simulink model "Control_test"  (R2014b)
settings: Solver=FixedStepDiscrete  StartTime=0.0  StopTime=Inf  FixedStep=0.001  RelTol=1e-3
PostLoadFcn:
  | , if any(exist('dsrtsu_mdlpostloadfcn', 'file') == [2, 3, 6]), try dsrtsu_mdlpostloadfcn('Execute', bdroot); catch fprintf('Error in PostLoadFcn (dsrtsu_mdlpostloadfcn) for model "%s":\n %s\n', bdroot, lasterr); end, end,
undefined symbols (not defined in the file or in its folder): dtLocal, slcm
libraries: rtican x163, simulink x14
(part 32 of 34)

== system Control_test/InputProcessing/VehicleCanProcessing/TCS3 ==
  Bus Creator : BusCreator  Inputs=17
  L_TCS3 : rtican/RTICAN Receive (RX)   Reserved1=[]  Reserved2=[]  Reserved3=[]  Reserved4=[]  SfcnMessage=[]  Msg_Struct=[]  BoardTypeNo=[]  BoardNo=[]  ChannelNo=[]  Parameters=[]  DialogFcn=[]  UnitName=[]  Revision=[]  UnitValues=[]  DSProperties=struct('RTI',struct('Version',uint32(5),'BlockType',struct('isSLSource',uint8(1),'isSLSink',uint8(1),'isHWSource',uint8(0),'isHWSink',uint8(0),'isSetup',uint8(0),'isInline',uint8(1),'isNonInline',uint8(0),'isInterrupt',uint8(0),'isChannelwise',uint8(0)),'IOBoardType','RTICAN','UnitType','MESSAGE','Identifier','RX','DialogType','MSVC','BlockSet','RTICAN','SlaveProcessor','CAN'))  RTIBlockInterface=struct('OutputPortsWidth',int32([1 1 1 1 1 1 1 1 1 1 1 1 1 1 1 1 1]),'OutputPortsActive',[1 1 1 1 1 1 1 1 1 1 1 1 1 1 1 1 1],'OutputPortsName',{{'aBasis','BrakeLight','DCEnable','AliveCounterTCS','MinGear','MaxGear','ACCReqLim','TQI_ACC','ACCEL_REF_ACC','ACCEnable','DriverOverride','StandStill','CheckSum_TCS3','ACC_EQUIP','PBRAKE_ACT','ACC_REQ','DriverBraking'}},'OutputPortsDataType',{{'SS_DOUBLE','SS_DOUBLE','SS_DOUBLE','SS_DOUBLE','SS_DOUBLE','SS_DOUBLE','SS_DOUBLE','SS_DOUBLE','SS_DOUBLE','SS_DOUBLE','SS_DOUBLE','SS_DOUBLE','SS_DOUBLE','SS_DOUBLE','SS_DOUBLE','SS_DOUBLE','SS_DOUBLE'}},'OutputPortsLabel',{{'aBasis','BrakeLight','DCEnable','AliveCounterTCS','MinGear','MaxGear','ACCReqLim','TQI_ACC','ACCEL_REF_ACC','ACCEnable','DriverOverride','StandStill','CheckSum_TCS3','ACC_EQUIP','PBRAKE_ACT','ACC_REQ','DriverBraking'}},'OutputPortsLabelMode','ON','InputPortsWidth',int32(0),'InputPortsActive',0,'DialogFcn','rtican_message_interface_gui','BlockDisplay',{{'','center'}},'IconTransparency','on','ParameterTunableNames',{{}},'InitLevel',3,'BlockName',struct('Token',{{'L_TCS3'}}),'SampleTime',{{-1}},'TriggerPort',{{'none'}},'EnablePort',{{'none'}})  RTIBlockParameters=struct('BoardTypeNo',{{1,'OFF',[]}},'BoardNo',{{1,'ON',[1 16]}},'ChannelNo',{{1,'ON',[1 2]}},'Parameters',{{struct('DataFileSupport',struct('DataFileSelectedMaster',1,'DataFileSelectedLocal',1,'DataFileName','c:\users\mpc_car\documents\github\mpc-car\controller\dbcfiles\hmc_can_for_ucb_v2.dbc|','DataFileDate',['21-Nov-2014 13:30:51'],'SelectedFile','c:\users\mpc_car\documents\github\mpc-car\dbcfiles\hmc_can_for_ucb_v2.dbc','InterfaceFcn','rtican_dbc_file_parser'),'Options',struct('StatusSelected',0,'TimeSelected',0,'DeltaTimeSelected',0,'BytePortSelected',0,'MessageLengthSelected',0,'TriggerPort',struct('Selected',0,'TriggerType',0),'UserCoding',struct('Selected',0,'InterfaceFile','UserDecodingFile','FcnName','UserDecodeFcn','InportSelected',0,'InportWidth',1,'OutportSelected',0,'OutportWidth',1),'EnablePortSelected',0,'SignalOnPortnameSelected',1,'UseRXService',0),'Message',struct('MsgOnBlocknameSelected',1,'MsgName','L_TCS3','MsgIdFormat',0,'MsgId',1072,'MsgLength',8,'NumSignals',17,'SampleTime',-1,'Signal',struct('SgnName',{'aBasis','BrakeLight','DCEnable','AliveCounterTCS','MinGear','MaxGear','ACCReqLim','TQI_ACC','ACCEL_REF_ACC','ACCEnable','DriverOverride','StandStill','CheckSum_TCS3','ACC_EQUIP','PBRAKE_ACT','ACC_REQ','DriverBraking'},'SgnStartBit',{0,11,12,13,16,19,22,24,32,43,45,47,48,52,53,54,55},'SgnLength',{11,1,1,3,3,3,2,8,11,2,2,1,4,1,1,1,1},'ByteLayout',{0,0,0,0,0,0,0,0,0,0,0,0,0,0,0,0,0},'Factor',{0.01,1,1,1,1,1,1,0.390625,0.01,1,1,1,1,1,1,1,1},'Offset',{-10.23,0,0,0,0,0,0,0,-10.23,0,0,0,0,0,0,0,0},'SgnComment',{'','','','','','','','','','','','','','','','',''},'SgnUnit',{'m/s^2','','','','','','','%','m/s^2','','','','','','','',''},'Min',{-10.23,0,0,0,0,0,0,0,-10.23,0,0,0,0,0,0,0,0},'Max',{10.24,1,1,7,7,7,3,99.609375,10.24,3,3,1,15,1,1,1,1},'SgnType',{0,0,0,0,0,0,0,0,0,0,0,0,0,0,0,0,0},'SLDataType',{'SS_DOUBLE','SS_DOUBLE','SS_DOUBLE','SS_DOUBLE','SS_DOUBLE','SS_DOUBLE','SS_DOUBLE','SS_DOUBLE','SS_DOUBLE','SS_DOUBLE','SS_DOUBLE','SS_DOUBLE','SS_DOUBLE','SS_DOUBLE','SS_DOUBLE','SS_DOUBLE','SS_DOUBLE'},'DataType',{0,0,0,0,0,0,1,0,0,0,0,0,0,0,0,0,0},'ModeValue',{-1,-1,-1,-1,-1,-1,-1,-1,-1,-1,-1,-1,-1,-1,-1,-1,-1}),'MsgIdNumFormat',0,'MsgComment',{{''}}),'Version',1.2,'general',struct('isFromLib',0)),'OFF',[]}},'GroupId',{{struct('Group',{{'RTICAN'}},'No',1,'Behavior',{{'NAMECHANGE'}},'BlockType',{{'SINK'}},'NameChangeFlag',0),'OFF',[]}},'SFcnRTICANMessage',{{struct('MsgType','RX','SFcnPortType','Scalar','MsgName','L_TCS3','MsgIdFormat','STD','MsgId',1072,'MsgLength',8,'NumSignals',17,'SampleTime',-1,'Signal',struct('SgnName',{'aBasis','BrakeLight','DCEnable','AliveCounterTCS','MinGear','MaxGear','ACCReqLim','TQI_ACC','ACCEL_REF_ACC','ACCEnable','DriverOverride','StandStill','CheckSum_TCS3','ACC_EQUIP','PBRAKE_ACT','ACC_REQ','DriverBraking'},'SgnStartBit',{0,11,12,13,16,19,22,24,32,43,45,47,48,52,53,54,55},'SgnLength',{11,1,1,3,3,3,2,8,11,2,2,1,4,1,1,1,1},'ByteLayout',{['little endian'],['little endian'],['little endian'],['little endian'],['little endian'],['little endian'],['little endian'],['little endian'],['little endian'],['little endian'],['little endian'],['little endian'],['little endian'],['little endian'],['little endian'],['little endian'],['little endian']},'Factor',{0.01,1,1,1,1,1,1,0.390625,0.01,1,1,1,1,1,1,1,1},'Offset',{-10.23,0,0,0,0,0,0,0,-10.23,0,0,0,0,0,0,0,0},'SgnType',{'standard','standard','standard','standard','standard','standard','standard','standard','standard','standard','standard','standard','standard','standard','standard','standard','standard'},'SLDataType',{'SS_DOUBLE','SS_DOUBLE','SS_DOUBLE','SS_DOUBLE','SS_DOUBLE','SS_DOUBLE','SS_DOUBLE','SS_DOUBLE','SS_DOUBLE','SS_DOUBLE','SS_DOUBLE','SS_DOUBLE','SS_DOUBLE','SS_DOUBLE','SS_DOUBLE','SS_DOUBLE','SS_DOUBLE'},'DataType',{['unsigned int'],['unsigned int'],['unsigned int'],['unsigned int'],['unsigned int'],['unsigned int'],['signed int'],['unsigned int'],['unsigned int'],['unsigned int'],['unsigned int'],['unsigned int'],['unsigned int'],['unsigned int'],['unsigned int'],['unsigned int'],['unsigned int']},'ModeValue',{-1,-1,-1,-1,-1,-1,-1,-1,-1,-1,-1,-1,-1,-1,-1,-1,-1}),'StatusSelected','no','TimeSelected','no','DeltaTimeSelected','no','BytePortSelected','no','MessageLengthSelected','no','TriggerPort',struct('Selected','no','TriggerType',0),'UserCoding',struct('Selected','no','InterfaceFile','UserDecodingFile','FcnName','UserDecodeFcn','InportSelected','no','InportWidth',1,'OutportSelected','no','OutportWidth',1),'EnablePortSelected','no','UseRXService','no','BoardType','DS1','BoardNo',1,'ControllerNo',1),'OFF',[]}},'TLCFileName',{{'rtican_rx_message','OFF',[]}})  RTISFcnParameters=struct('SFcnRTICANMessage','struct','TLCFileName','char')  RTIBlockParaDefault=struct('BoardTypeNo',4302,'BoardNo',1,'ChannelNo',1,'Parameters',struct('DataFileSupport',struct('DataFileSelectedMaster',0,'DataFileSelectedLocal',0,'DataFileName','','DataFileDate','','SelectedFile',['<no file selected>']),'Options',struct('StatusSelected',1,'TimeSelected',1,'DeltaTimeSelected',1,'BytePortSelected',0,'MessageLengthSelected',0,'TriggerPort',struct('Selected',0,'TriggerType','rising'),'UserCoding',struct('Selected',0,'InterfaceFile','UserDecodingFile','FcnName','UserDecodeFcn','InportSelected',0,'InportWidth',1,'OutportSelected',0,'OutportWidth',1),'EnablePortSelected',0,'SignalOnPortnameSelected',1,'UseRXService',0),'Message',struct('MsgOnBlocknameSelected',0,'MsgName',['RX Message'],'MsgIdFormat',0,'MsgId',100,'MsgLength',8,'NumSignals',1,'SampleTime',-1,'Signal',struct('SgnName',['RX signal'],'SgnStartBit',0,'SgnLength',8,'SgnType',0,'ModeValue',-1,'DataType',0,'SLDataType','SS_DOUBLE','ByteLayout',0,'Factor',1,'Offset',0,'Min',0,'Max',255,'SgnComment',{{}},'SgnUnit',''),'MsgIdNumFormat',0,'MsgComment',{{''}}),'Version',1.2,'general',struct('isFromLib',1)),'GroupId',struct('Group',{{'RTICAN'}},'No',1,'Behavior',{{'NAMECHANGE'}},'BlockType',{{'SINK'}},'NameChangeFlag',0),'SFcnRTICANMessage',struct('MsgType','RX','MsgName',['RX Message'],'MsgIdFormat','STD','MsgId',100,'MsgLength',8,'NumSignals',1,'SampleTime',-1,'Signal',struct('SgnName',['RX signal'],'SgnStartBit',0,'SgnLength',8,'SgnType','standard','ModeValue',-1,'DataType',['unsigned int'],'ByteLayout',['little endian'],'SLDataType','SS_DOUBLE','Factor',1,'Offset',0),'StatusSelected','yes','TimeSelected','yes','DeltaTimeSelected','yes','BytePortSelected','no','MessageLengthSelected','no','EnablePortSelected','no','UserCoding',struct('Selected','no','InterfaceFile','UserDecodingFile','FcnName','UserDecodeFcn','InportSelected','no','InportWidth',1,'OutportSelected','no','OutportWidth',1),'TriggerPort',struct('Selected','no','TriggerType','rising'),'UseRXService','no','BoardType','DS4302','BoardNo',1,'ControllerNo',1,'SFcnPortType','Scalar'),'TLCFileName','rtican_rx_message')
      settings: AttributesFormatString=Group Id: RTICAN1\n
  TCS3_CAN : Outport
  wires:
  Bus Creator/1 -> TCS3_CAN/1  "TCS3_CAN"
  L_TCS3/1 -> Bus Creator/1  "aBasis"
  L_TCS3/2 -> Bus Creator/2  "BrakeLight"
  L_TCS3/3 -> Bus Creator/3  "DCEnable"
  L_TCS3/4 -> Bus Creator/4  "AliveCounterTCS"
  L_TCS3/5 -> Bus Creator/5  "MinGear"
  L_TCS3/6 -> Bus Creator/6  "MaxGear"
  L_TCS3/7 -> Bus Creator/7  "ACCReqLim"
  L_TCS3/8 -> Bus Creator/8  "TQI_ACC"
  L_TCS3/9 -> Bus Creator/9  "ACCEL_REF_ACC"
  L_TCS3/10 -> Bus Creator/10  "ACCEnable"
  L_TCS3/11 -> Bus Creator/11  "DriverOverride"
  L_TCS3/12 -> Bus Creator/12  "StandStill"
  L_TCS3/13 -> Bus Creator/13  "CheckSum_TCS3"
  L_TCS3/14 -> Bus Creator/14  "ACC_EQUIP"
  L_TCS3/15 -> Bus Creator/15  "PBRAKE_ACT"
  L_TCS3/16 -> Bus Creator/16  "ACC_REQ"
  L_TCS3/17 -> Bus Creator/17  "DriverBraking"

== system Control_test/InputProcessing/VehicleCanProcessing/TCS3Processing ==
  In1 : Inport
  Bus Creator9 : BusCreator  Inputs=12
  Bus Selector9 : BusSelector  OutputSignals=aBasis,DCEnable,ACCReqLim,TQI_ACC,ACCEL_REF_ACC,ACCEnable,DriverOverride,StandStill,PBRAKE_ACT,ACC_REQ,ACC_EQUIP,DriverBraking
  Out1 : Outport
  wires:
  In1/1 -> Bus Selector9/1
  Bus Creator9/1 -> Out1/1  "TCS3Data"
  Bus Selector9/2 -> Bus Creator9/2  "<DCEnable>"
  Bus Selector9/1 -> Bus Creator9/1  "<aBasis>"
  Bus Selector9/3 -> Bus Creator9/3  "<ACCReqLim>"
  Bus Selector9/4 -> Bus Creator9/4  "<TQI_ACC>"
  Bus Selector9/5 -> Bus Creator9/5  "<ACCEL_REF_ACC>"
  Bus Selector9/6 -> Bus Creator9/6  "<ACCEnable>"
  Bus Selector9/7 -> Bus Creator9/7  "<DriverOverride>"
  Bus Selector9/8 -> Bus Creator9/8  "<StandStill>"
  Bus Selector9/9 -> Bus Creator9/9  "<PBRAKE_ACT>"
  Bus Selector9/10 -> Bus Creator9/10  "<ACC_REQ>"
  Bus Selector9/11 -> Bus Creator9/11  "<ACC_EQUIP>"
  Bus Selector9/12 -> Bus Creator9/12  "<DriverBraking>"

== system Control_test/InputProcessing/VehicleCanProcessing/TCU1 ==
  Bus Creator : BusCreator  Inputs=14
  L_TCU1 : rtican/RTICAN Receive (RX)   Reserved1=[]  Reserved2=[]  Reserved3=[]  Reserved4=[]  SfcnMessage=[]  Msg_Struct=[]  BoardTypeNo=[]  BoardNo=[]  ChannelNo=[]  Parameters=[]  DialogFcn=[]  UnitName=[]  Revision=[]  UnitValues=[]  DSProperties=struct('RTI',struct('Version',uint32(5),'BlockType',struct('isSLSource',uint8(1),'isSLSink',uint8(1),'isHWSource',uint8(0),'isHWSink',uint8(0),'isSetup',uint8(0),'isInline',uint8(1),'isNonInline',uint8(0),'isInterrupt',uint8(0),'isChannelwise',uint8(0)),'IOBoardType','RTICAN','UnitType','MESSAGE','Identifier','RX','DialogType','MSVC','BlockSet','RTICAN','SlaveProcessor','CAN'))  RTIBlockInterface=struct('OutputPortsWidth',int32([1 1 1 1 1 1 1 1 1 1 1 1 1 1]),'OutputPortsActive',[1 1 1 1 1 1 1 1 1 1 1 1 1 1],'OutputPortsName',{{'SWI_GS','GEAR_TYPE','TCU_TYPE','F_OBD','G_SEL_DISP','TCU_OBD','TQI_TCU','TEMP_AT','N_TC','TQI_TCU_INC','F_TCU','SWI_CC','TCU_STAT','TAR_GC'}},'OutputPortsDataType',{{'SS_DOUBLE','SS_DOUBLE','SS_DOUBLE','SS_DOUBLE','SS_DOUBLE','SS_DOUBLE','SS_DOUBLE','SS_DOUBLE','SS_DOUBLE','SS_DOUBLE','SS_DOUBLE','SS_DOUBLE','SS_DOUBLE','SS_DOUBLE'}},'OutputPortsLabel',{{'SWI_GS','GEAR_TYPE','TCU_TYPE','F_OBD','G_SEL_DISP','TCU_OBD','TQI_TCU','TEMP_AT','N_TC','TQI_TCU_INC','F_TCU','SWI_CC','TCU_STAT','TAR_GC'}},'OutputPortsLabelMode','ON','InputPortsWidth',int32(0),'InputPortsActive',0,'DialogFcn','rtican_message_interface_gui','BlockDisplay',{{'','center'}},'IconTransparency','on','ParameterTunableNames',{{}},'InitLevel',3,'BlockName',struct('Token',{{'L_TCU1'}}),'SampleTime',{{-1}},'TriggerPort',{{'none'}},'EnablePort',{{'none'}})  RTIBlockParameters=struct('BoardTypeNo',{{1,'OFF',[]}},'BoardNo',{{1,'ON',[1 16]}},'ChannelNo',{{1,'ON',[1 2]}},'Parameters',{{struct('DataFileSupport',struct('DataFileSelectedMaster',1,'DataFileSelectedLocal',1,'DataFileName','c:\users\mpc_car\documents\github\mpc-car\controller\dbcfiles\hmc_can_for_ucb_v1.dbc|','DataFileDate',['21-Nov-2014 13:30:51'],'SelectedFile','c:\users\mpc_car\documents\github\mpc-car\dbcfiles\hmc_can_for_ucb_v2.dbc','InterfaceFcn','rtican_dbc_file_parser'),'Options',struct('StatusSelected',0,'TimeSelected',0,'DeltaTimeSelected',0,'BytePortSelected',0,'MessageLengthSelected',0,'TriggerPort',struct('Selected',0,'TriggerType',0),'UserCoding',struct('Selected',0,'InterfaceFile','UserDecodingFile','FcnName','UserDecodeFcn','InportSelected',0,'InportWidth',1,'OutportSelected',0,'OutportWidth',1),'EnablePortSelected',0,'SignalOnPortnameSelected',1,'UseRXService',0),'Message',struct('MsgOnBlocknameSelected',1,'MsgName','L_TCU1','MsgIdFormat',0,'MsgId',1087,'MsgLength',8,'NumSignals',14,'SampleTime',-1,'Signal',struct('SgnName',{'SWI_GS','GEAR_TYPE','TCU_TYPE','F_OBD','G_SEL_DISP','TCU_OBD','TQI_TCU','TEMP_AT','N_TC','TQI_TCU_INC','F_TCU','SWI_CC','TCU_STAT','TAR_GC'},'SgnStartBit',{0,1,5,7,8,12,16,24,32,48,56,58,60,61},'SgnLength',{1,4,2,1,4,4,8,8,16,8,2,2,1,3},'ByteLayout',{0,0,0,0,0,0,0,0,0,0,0,0,0,0},'Factor',{1,1,1,1,1,1,0.390625,1,0.25,0.390625,1,1,1,1},'Offset',{0,0,0,0,0,0,0,-40,0,0,0,0,0,0},'SgnComment',{'','','','','','','','','','','','','',''},'SgnUnit',{'','','','','','','%','¡É','rpm','%','','','',''},'Min',{0,0,0,0,0,0,0,-40,0,0,0,0,0,0},'Max',{1,15,3,1,15,15,99.609375,214,16383.5,99.609375,3,3,1,7},'SgnType',{0,0,0,0,0,0,0,0,0,0,0,0,0,0},'SLDataType',{'SS_DOUBLE','SS_DOUBLE','SS_DOUBLE','SS_DOUBLE','SS_DOUBLE','SS_DOUBLE','SS_DOUBLE','SS_DOUBLE','SS_DOUBLE','SS_DOUBLE','SS_DOUBLE','SS_DOUBLE','SS_DOUBLE','SS_DOUBLE'},'DataType',{0,0,0,0,0,0,0,0,0,0,0,0,0,0},'ModeValue',{-1,-1,-1,-1,-1,-1,-1,-1,-1,-1,-1,-1,-1,-1}),'MsgIdNumFormat',0,'MsgComment',{{''}}),'Version',1.2,'general',struct('isFromLib',0)),'OFF',[]}},'GroupId',{{struct('Group',{{'RTICAN'}},'No',1,'Behavior',{{'NAMECHANGE'}},'BlockType',{{'SINK'}},'NameChangeFlag',0),'OFF',[]}},'SFcnRTICANMessage',{{struct('MsgType','RX','SFcnPortType','Scalar','MsgName','L_TCU1','MsgIdFormat','STD','MsgId',1087,'MsgLength',8,'NumSignals',14,'SampleTime',-1,'Signal',struct('SgnName',{'SWI_GS','GEAR_TYPE','TCU_TYPE','F_OBD','G_SEL_DISP','TCU_OBD','TQI_TCU','TEMP_AT','N_TC','TQI_TCU_INC','F_TCU','SWI_CC','TCU_STAT','TAR_GC'},'SgnStartBit',{0,1,5,7,8,12,16,24,32,48,56,58,60,61},'SgnLength',{1,4,2,1,4,4,8,8,16,8,2,2,1,3},'ByteLayout',{['little endian'],['little endian'],['little endian'],['little endian'],['little endian'],['little endian'],['little endian'],['little endian'],['little endian'],['little endian'],['little endian'],['little endian'],['little endian'],['little endian']},'Factor',{1,1,1,1,1,1,0.390625,1,0.25,0.390625,1,1,1,1},'Offset',{0,0,0,0,0,0,0,-40,0,0,0,0,0,0},'SgnType',{'standard','standard','standard','standard','standard','standard','standard','standard','standard','standard','standard','standard','standard','standard'},'SLDataType',{'SS_DOUBLE','SS_DOUBLE','SS_DOUBLE','SS_DOUBLE','SS_DOUBLE','SS_DOUBLE','SS_DOUBLE','SS_DOUBLE','SS_DOUBLE','SS_DOUBLE','SS_DOUBLE','SS_DOUBLE','SS_DOUBLE','SS_DOUBLE'},'DataType',{['unsigned int'],['unsigned int'],['unsigned int'],['unsigned int'],['unsigned int'],['unsigned int'],['unsigned int'],['unsigned int'],['unsigned int'],['unsigned int'],['unsigned int'],['unsigned int'],['unsigned int'],['unsigned int']},'ModeValue',{-1,-1,-1,-1,-1,-1,-1,-1,-1,-1,-1,-1,-1,-1}),'StatusSelected','no','TimeSelected','no','DeltaTimeSelected','no','BytePortSelected','no','MessageLengthSelected','no','TriggerPort',struct('Selected','no','TriggerType',0),'UserCoding',struct('Selected','no','InterfaceFile','UserDecodingFile','FcnName','UserDecodeFcn','InportSelected','no','InportWidth',1,'OutportSelected','no','OutportWidth',1),'EnablePortSelected','no','UseRXService','no','BoardType','DS1','BoardNo',1,'ControllerNo',1),'OFF',[]}},'TLCFileName',{{'rtican_rx_message','OFF',[]}})  RTISFcnParameters=struct('SFcnRTICANMessage','struct','TLCFileName','char')  RTIBlockParaDefault=struct('BoardTypeNo',4302,'BoardNo',1,'ChannelNo',1,'Parameters',struct('DataFileSupport',struct('DataFileSelectedMaster',0,'DataFileSelectedLocal',0,'DataFileName','','DataFileDate','','SelectedFile',['<no file selected>']),'Options',struct('StatusSelected',1,'TimeSelected',1,'DeltaTimeSelected',1,'BytePortSelected',0,'MessageLengthSelected',0,'TriggerPort',struct('Selected',0,'TriggerType','rising'),'UserCoding',struct('Selected',0,'InterfaceFile','UserDecodingFile','FcnName','UserDecodeFcn','InportSelected',0,'InportWidth',1,'OutportSelected',0,'OutportWidth',1),'EnablePortSelected',0,'SignalOnPortnameSelected',1,'UseRXService',0),'Message',struct('MsgOnBlocknameSelected',0,'MsgName',['RX Message'],'MsgIdFormat',0,'MsgId',100,'MsgLength',8,'NumSignals',1,'SampleTime',-1,'Signal',struct('SgnName',['RX signal'],'SgnStartBit',0,'SgnLength',8,'SgnType',0,'ModeValue',-1,'DataType',0,'SLDataType','SS_DOUBLE','ByteLayout',0,'Factor',1,'Offset',0,'Min',0,'Max',255,'SgnComment',{{}},'SgnUnit',''),'MsgIdNumFormat',0,'MsgComment',{{''}}),'Version',1.2,'general',struct('isFromLib',1)),'GroupId',struct('Group',{{'RTICAN'}},'No',1,'Behavior',{{'NAMECHANGE'}},'BlockType',{{'SINK'}},'NameChangeFlag',0),'SFcnRTICANMessage',struct('MsgType','RX','MsgName',['RX Message'],'MsgIdFormat','STD','MsgId',100,'MsgLength',8,'NumSignals',1,'SampleTime',-1,'Signal',struct('SgnName',['RX signal'],'SgnStartBit',0,'SgnLength',8,'SgnType','standard','ModeValue',-1,'DataType',['unsigned int'],'ByteLayout',['little endian'],'SLDataType','SS_DOUBLE','Factor',1,'Offset',0),'StatusSelected','yes','TimeSelected','yes','DeltaTimeSelected','yes','BytePortSelected','no','MessageLengthSelected','no','EnablePortSelected','no','UserCoding',struct('Selected','no','InterfaceFile','UserDecodingFile','FcnName','UserDecodeFcn','InportSelected','no','InportWidth',1,'OutportSelected','no','OutportWidth',1),'TriggerPort',struct('Selected','no','TriggerType','rising'),'UseRXService','no','BoardType','DS4302','BoardNo',1,'ControllerNo',1,'SFcnPortType','Scalar'),'TLCFileName','rtican_rx_message')
      settings: AttributesFormatString=Group Id: RTICAN1\n
  TCU1_CAN : Outport
  wires:
  Bus Creator/1 -> TCU1_CAN/1  "TCU1_CAN"
  L_TCU1/1 -> Bus Creator/1  "SWI_GS"
  L_TCU1/2 -> Bus Creator/2  "GEAR_TYPE"
  L_TCU1/3 -> Bus Creator/3  "TCU_TYPE"
  L_TCU1/4 -> Bus Creator/4  "F_OBD"
  L_TCU1/7 -> Bus Creator/5  "TQI_TCU"
  L_TCU1/5 -> Bus Creator/6  "G_SEL_DISP"
  L_TCU1/6 -> Bus Creator/7  "TCU_OBD"
  L_TCU1/8 -> Bus Creator/8  "TEMP_AT"
  L_TCU1/9 -> Bus Creator/9  "N_TC"
  L_TCU1/10 -> Bus Creator/10  "TQI_TCU_INC"
  L_TCU1/11 -> Bus Creator/11  "F_TCU"
  L_TCU1/12 -> Bus Creator/12  "SWI_CC"
  L_TCU1/13 -> Bus Creator/13  "TCU_STAT"
  L_TCU1/14 -> Bus Creator/14  "TAR_GC"

== system Control_test/InputProcessing/VehicleCanProcessing/TCU1Processing ==
  In1 : Inport
  Bus Creator9 : BusCreator  Inputs=7
  Bus Selector9 : BusSelector  OutputSignals=TAR_GC,F_TCU,N_TC,SWI_GS,SWI_CC,G_SEL_DISP
  TCU1 Processing : Subsystem
  Out1 : Outport
  wires:
  Bus Selector9/1 -> TCU1 Processing/1(TAR_GC_CAN)  "<TAR_GC>"
  Bus Selector9/2 -> TCU1 Processing/2(F_TCU_CAN)  "<F_TCU>"
  Bus Selector9/3 -> TCU1 Processing/3(N_TC_CAN)  "<N_TC>"
  Bus Selector9/4 -> TCU1 Processing/4(SWI_GS_CAN)  "<SWI_GS>"
  Bus Selector9/5 -> TCU1 Processing/5(SWI_CC_CAN)  "<SWI_CC>"
  Bus Selector9/6 -> TCU1 Processing/6(G_SEL_DISP_CAN)  "<G_SEL_DISP>"
  TCU1 Processing/1(ipTargetGear) -> Bus Creator9/1
  TCU1 Processing/2(ipTcuFail) -> Bus Creator9/2
  TCU1 Processing/3(ipTubSpd [rpm]) -> Bus Creator9/3
  TCU1 Processing/4(ipGearChange) -> Bus Creator9/4
  TCU1 Processing/5(ipLockupClutch) -> Bus Creator9/5
  TCU1 Processing/6(ipSftLvrPos) -> Bus Creator9/6
  TCU1 Processing/7(ipSftLvrDFlag) -> Bus Creator9/7
  Bus Creator9/1 -> Out1/1  "TCU1Data"
  In1/1 -> Bus Selector9/1

== system Control_test/InputProcessing/VehicleCanProcessing/WHL_SPD ==
  Bus Creator : BusCreator
  L_WHL_SPD : rtican/RTICAN Receive (RX)   Reserved1=[]  Reserved2=[]  Reserved3=[]  Reserved4=[]  SfcnMessage=[]  Msg_Struct=[]  BoardTypeNo=[]  BoardNo=[]  ChannelNo=[]  Parameters=[]  DialogFcn=[]  UnitName=[]  Revision=[]  UnitValues=[]  DSProperties=struct('RTI',struct('Version',uint32(5),'BlockType',struct('isSLSource',uint8(1),'isSLSink',uint8(1),'isHWSource',uint8(0),'isHWSink',uint8(0),'isSetup',uint8(0),'isInline',uint8(1),'isNonInline',uint8(0),'isInterrupt',uint8(0),'isChannelwise',uint8(0)),'IOBoardType','RTICAN','UnitType','MESSAGE','Identifier','RX','DialogType','MSVC','BlockSet','RTICAN','SlaveProcessor','CAN'))  RTIBlockInterface=struct('OutputPortsWidth',int32([1 1 1 1]),'OutputPortsActive',[1 1 1 1],'OutputPortsName',{{'WHL_SPD_FL','WHL_SPD_RR','WHL_SPD_FR','WHL_SPD_RL'}},'OutputPortsDataType',{{'SS_DOUBLE','SS_DOUBLE','SS_DOUBLE','SS_DOUBLE'}},'OutputPortsLabel',{{'WHL_SPD_FL','WHL_SPD_RR','WHL_SPD_FR','WHL_SPD_RL'}},'OutputPortsLabelMode','ON','InputPortsWidth',int32(0),'InputPortsActive',0,'DialogFcn','rtican_message_interface_gui','BlockDisplay',{{'','center'}},'IconTransparency','on','ParameterTunableNames',{{}},'InitLevel',3,'BlockName',struct('Token',{{'L_WHL_SPD'}}),'SampleTime',{{-1}},'TriggerPort',{{'none'}},'EnablePort',{{'none'}})  RTIBlockParameters=struct('BoardTypeNo',{{1,'OFF',[]}},'BoardNo',{{1,'ON',[1 16]}},'ChannelNo',{{1,'ON',[1 2]}},'Parameters',{{struct('DataFileSupport',struct('DataFileSelectedMaster',1,'DataFileSelectedLocal',1,'DataFileName','c:\users\mpc_car\documents\github\mpc-car\controller\dbcfiles\hmc_can_for_ucb_v1.dbc|','DataFileDate',['21-Nov-2014 13:30:51'],'SelectedFile','c:\users\mpc_car\documents\github\mpc-car\dbcfiles\hmc_can_for_ucb_v2.dbc','InterfaceFcn','rtican_dbc_file_parser'),'Options',struct('StatusSelected',0,'TimeSelected',0,'DeltaTimeSelected',0,'BytePortSelected',0,'MessageLengthSelected',0,'TriggerPort',struct('Selected',0,'TriggerType',0),'UserCoding',struct('Selected',0,'InterfaceFile','UserDecodingFile','FcnName','UserDecodeFcn','InportSelected',0,'InportWidth',1,'OutportSelected',0,'OutportWidth',1),'EnablePortSelected',0,'SignalOnPortnameSelected',1,'UseRXService',0),'Message',struct('MsgOnBlocknameSelected',1,'MsgName','L_WHL_SPD','MsgIdFormat',0,'MsgId',522,'MsgLength',8,'NumSignals',4,'SampleTime',-1,'Signal',struct('SgnName',{'WHL_SPD_FL','WHL_SPD_RR','WHL_SPD_FR','WHL_SPD_RL'},'SgnStartBit',{0,16,32,48},'SgnLength',{14,14,14,14},'ByteLayout',{0,0,0,0},'Factor',{0.03125,0.03125,0.03125,0.03125},'Offset',{0,0,0,0},'SgnComment',{['This signal is for the SCC system and higher reolution of wheel speed signal.'],['This signal is for the SCC system and higher reolution of wheel speed signal.'],['This signal is for the SCC system and higher reolution of wheel speed signal.'],['This signal is for the SCC system and higher reolution of wheel speed signal.']},'SgnUnit',{'km/h','km/h','km/h','km/h'},'Min',{0,0,0,0},'Max',{511.96875,511.96875,511.96875,511.96875},'SgnType',{0,0,0,0},'SLDataType',{'SS_DOUBLE','SS_DOUBLE','SS_DOUBLE','SS_DOUBLE'},'DataType',{0,0,0,0},'ModeValue',{-1,-1,-1,-1}),'MsgIdNumFormat',0,'MsgComment',{{''}}),'Version',1.2,'general',struct('isFromLib',0)),'OFF',[]}},'GroupId',{{struct('Group',{{'RTICAN'}},'No',1,'Behavior',{{'NAMECHANGE'}},'BlockType',{{'SINK'}},'NameChangeFlag',0),'OFF',[]}},'SFcnRTICANMessage',{{struct('MsgType','RX','SFcnPortType','Scalar','MsgName','L_WHL_SPD','MsgIdFormat','STD','MsgId',522,'MsgLength',8,'NumSignals',4,'SampleTime',-1,'Signal',struct('SgnName',{'WHL_SPD_FL','WHL_SPD_RR','WHL_SPD_FR','WHL_SPD_RL'},'SgnStartBit',{0,16,32,48},'SgnLength',{14,14,14,14},'ByteLayout',{['little endian'],['little endian'],['little endian'],['little endian']},'Factor',{0.03125,0.03125,0.03125,0.03125},'Offset',{0,0,0,0},'SgnType',{'standard','standard','standard','standard'},'SLDataType',{'SS_DOUBLE','SS_DOUBLE','SS_DOUBLE','SS_DOUBLE'},'DataType',{['unsigned int'],['unsigned int'],['unsigned int'],['unsigned int']},'ModeValue',{-1,-1,-1,-1}),'StatusSelected','no','TimeSelected','no','DeltaTimeSelected','no','BytePortSelected','no','MessageLengthSelected','no','TriggerPort',struct('Selected','no','TriggerType',0),'UserCoding',struct('Selected','no','InterfaceFile','UserDecodingFile','FcnName','UserDecodeFcn','InportSelected','no','InportWidth',1,'OutportSelected','no','OutportWidth',1),'EnablePortSelected','no','UseRXService','no','BoardType','DS1','BoardNo',1,'ControllerNo',1),'OFF',[]}},'TLCFileName',{{'rtican_rx_message','OFF',[]}})  RTISFcnParameters=struct('SFcnRTICANMessage','struct','TLCFileName','char')  RTIBlockParaDefault=struct('BoardTypeNo',4302,'BoardNo',1,'ChannelNo',1,'Parameters',struct('DataFileSupport',struct('DataFileSelectedMaster',0,'DataFileSelectedLocal',0,'DataFileName','','DataFileDate','','SelectedFile',['<no file selected>']),'Options',struct('StatusSelected',1,'TimeSelected',1,'DeltaTimeSelected',1,'BytePortSelected',0,'MessageLengthSelected',0,'TriggerPort',struct('Selected',0,'TriggerType','rising'),'UserCoding',struct('Selected',0,'InterfaceFile','UserDecodingFile','FcnName','UserDecodeFcn','InportSelected',0,'InportWidth',1,'OutportSelected',0,'OutportWidth',1),'EnablePortSelected',0,'SignalOnPortnameSelected',1,'UseRXService',0),'Message',struct('MsgOnBlocknameSelected',0,'MsgName',['RX Message'],'MsgIdFormat',0,'MsgId',100,'MsgLength',8,'NumSignals',1,'SampleTime',-1,'Signal',struct('SgnName',['RX signal'],'SgnStartBit',0,'SgnLength',8,'SgnType',0,'ModeValue',-1,'DataType',0,'SLDataType','SS_DOUBLE','ByteLayout',0,'Factor',1,'Offset',0,'Min',0,'Max',255,'SgnComment',{{}},'SgnUnit',''),'MsgIdNumFormat',0,'MsgComment',{{''}}),'Version',1.2,'general',struct('isFromLib',1)),'GroupId',struct('Group',{{'RTICAN'}},'No',1,'Behavior',{{'NAMECHANGE'}},'BlockType',{{'SINK'}},'NameChangeFlag',0),'SFcnRTICANMessage',struct('MsgType','RX','MsgName',['RX Message'],'MsgIdFormat','STD','MsgId',100,'MsgLength',8,'NumSignals',1,'SampleTime',-1,'Signal',struct('SgnName',['RX signal'],'SgnStartBit',0,'SgnLength',8,'SgnType','standard','ModeValue',-1,'DataType',['unsigned int'],'ByteLayout',['little endian'],'SLDataType','SS_DOUBLE','Factor',1,'Offset',0),'StatusSelected','yes','TimeSelected','yes','DeltaTimeSelected','yes','BytePortSelected','no','MessageLengthSelected','no','EnablePortSelected','no','UserCoding',struct('Selected','no','InterfaceFile','UserDecodingFile','FcnName','UserDecodeFcn','InportSelected','no','InportWidth',1,'OutportSelected','no','OutportWidth',1),'TriggerPort',struct('Selected','no','TriggerType','rising'),'UseRXService','no','BoardType','DS4302','BoardNo',1,'ControllerNo',1,'SFcnPortType','Scalar'),'TLCFileName','rtican_rx_message')
      settings: AttributesFormatString=Group Id: RTICAN1\n
  WHL_SPD_CAN : Outport
  wires:
  Bus Creator/1 -> WHL_SPD_CAN/1  "WHL_SPD_CAN"
  L_WHL_SPD/1 -> Bus Creator/1  "WHL_SPD_FL"
  L_WHL_SPD/2 -> Bus Creator/2  "WHL_SPD_RR"
  L_WHL_SPD/3 -> Bus Creator/3  "WHL_SPD_FR"
  L_WHL_SPD/4 -> Bus Creator/4  "WHL_SPD_RL"

== system Control_test/InputProcessing/VehicleCanProcessing/WhlSpdProcessing ==
  In1 : Inport
  Bus Creator2 : BusCreator  Inputs=10
  Bus Selector2 : BusSelector  OutputSignals=WHL_SPD_FL,WHL_SPD_FR,WHL_SPD_RL,WHL_SPD_RR
  WhlSpd Processing : Subsystem
  Out1 : Outport
  tag scope: ipVehSpd=global
  wires:
  Bus Creator2/1 -> Out1/1  "WhlSpdData"
  WhlSpd Processing/10(ipVehSpdWhl [m/s]) -> [ipVehSpd], Bus Creator2/10
  WhlSpd Processing/9(ipVehSpdWhl [kph]) -> Bus Creator2/9
  WhlSpd Processing/8(ipWhlSpdRrEr) -> Bus Creator2/8
  WhlSpd Processing/7(ipWhlSpdRr [kph]) -> Bus Creator2/7
  WhlSpd Processing/6(ipWhlSpdRlEr) -> Bus Creator2/6
  WhlSpd Processing/5(ipWhlSpdRl [kph]) -> Bus Creator2/5
  WhlSpd Processing/4(ipWhlSpdFrEr) -> Bus Creator2/4
  WhlSpd Processing/3(ipWhlSpdFr [kph]) -> Bus Creator2/3
  WhlSpd Processing/2(ipWhlSpdFlEr) -> Bus Creator2/2
  WhlSpd Processing/1(ipWhlSpdFl [kph]) -> Bus Creator2/1
  Bus Selector2/4 -> WhlSpd Processing/4(WHL_SPD_RR_CAN)  "<WHL_SPD_RR>"
  Bus Selector2/3 -> WhlSpd Processing/3(WHL_SPD_RL_CAN)  "<WHL_SPD_RL>"
  Bus Selector2/2 -> WhlSpd Processing/2(WHL_SPD_FR_CAN)  "<WHL_SPD_FR>"
  Bus Selector2/1 -> WhlSpd Processing/1(WHL_SPD_FL_CAN)  "<WHL_SPD_FL>"
  In1/1 -> Bus Selector2/1

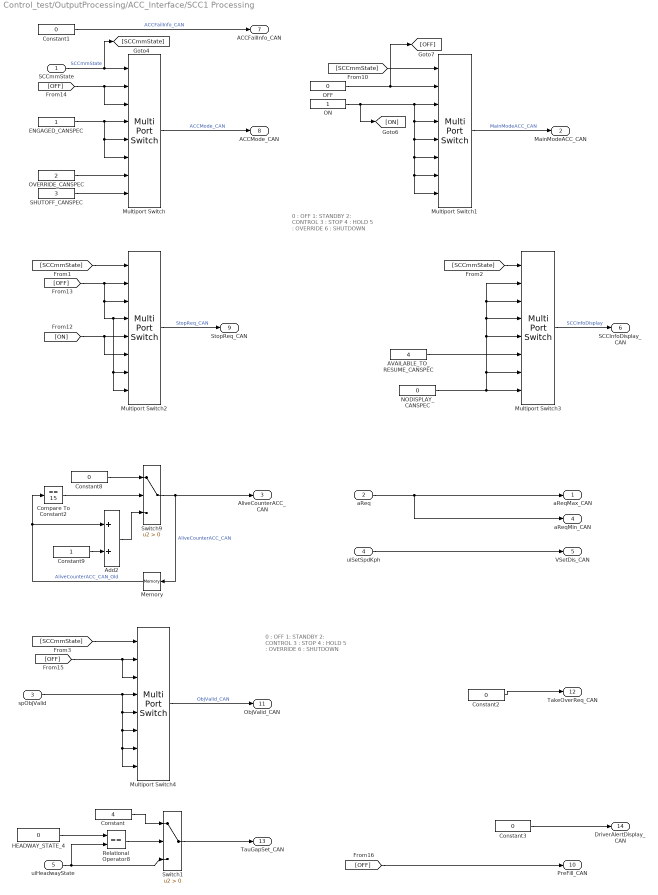
== system Control_test/OutputProcessing/ACC_Interface/SCC1 Processing ==
  note: 0 : OFF
      | 1: STANDBY
      | 2: CONTROL
      | 3 : STOP
      | 4 : HOLD
      | 5 : OVERRIDE
      | 6 : SHUTDOWN
  note: 0 : OFF
      | 1: STANDBY
      | 2: CONTROL
      | 3 : STOP
      | 4 : HOLD
      | 5 : OVERRIDE
      | 6 : SHUTDOWN
  SCCmmState : Inport
  aReq : Inport  Port=2
  spObjValid : Inport  Port=3
  uiSetSpdKph : Inport  Port=4
  uiHeadwayState : Inport  Port=5
  AVAILABLE_TO_RESUME_CANSPEC : Constant  Value=4  SampleTime=Inf
  Add2 : Sum
  Compare To Constant2 : simulink/Logic and Bit Operations/Compare To Constant  relop===  const=15  OutDataTypeStr=uint8  ZeroCross=off
  Constant : Constant  Value=4  SampleTime=Inf
  Constant{1..3,8} (4 alike) : Constant  Value=0  SampleTime=Inf
  Constant9 : Constant  SampleTime=Inf
  ENGAGED_CANSPEC : Constant  SampleTime=Inf
  HEADWAY_STATE_4 : Constant  Value=0  SampleTime=0.02
  Memory : Memory  InheritSampleTime=on
  Multiport Switch{,1..4} (5 alike) : MultiPortSwitch  DataPortOrder=Zero-based contiguous  Inputs=7  zeroidx=on
  NODISPLAY_CANSPEC : Constant  Value=0  SampleTime=Inf
  OFF : Constant  Value=0  SampleTime=Inf
  ON : Constant  SampleTime=Inf
  OVERRIDE_CANSPEC : Constant  Value=2  SampleTime=Inf
  Relational Operator8 : RelationalOperator  Operator===  OutDataTypeStr=boolean
  SHUTOFF_CANSPEC : Constant  Value=3  SampleTime=Inf
  Switch1 : Switch  Criteria=u2 > Threshold
  Switch9 : Switch  Criteria=u2 > Threshold
  aReqMax_CAN : Outport
  MainModeACC_CAN : Outport  Port=2
  AliveCounterACC_CAN : Outport  Port=3
  aReqMin_CAN : Outport  Port=4
  VSetDis_CAN : Outport  Port=5
  SCCInfoDisplay_CAN : Outport  Port=6
  ACCFailInfo_CAN : Outport  Port=7
  ACCMode_CAN : Outport  Port=8
  StopReq_CAN : Outport  Port=9
  PreFill_CAN : Outport  Port=10
  ObjValid_CAN : Outport  Port=11
  TakeOverReq_CAN : Outport  Port=12
  TauGapSet_CAN : Outport  Port=13
  DriverAlertDisplay_CAN : Outport  Port=14
  wires:
  Switch1/1 -> TauGapSet_CAN/1
  Constant/1 -> Switch1/1
  Relational Operator8/1 -> Switch1/2
  spObjValid/1 -> Multiport Switch4/8, Multiport Switch4/7, Multiport Switch4/6, Multiport Switch4/5, Multiport Switch4/4
  [OFF] -> Multiport Switch4/3, Multiport Switch4/2
  [SCCmmState] -> Multiport Switch4/1
  uiSetSpdKph/1 -> VSetDis_CAN/1
  Multiport Switch3/1 -> SCCInfoDisplay_CAN/1  "SCCInfoDisplay"
  AVAILABLE_TO_RESUME_CANSPEC/1 -> Multiport Switch3/6
  [SCCmmState] -> Multiport Switch3/1
  Multiport Switch2/1 -> StopReq_CAN/1  "StopReq_CAN"
  [OFF] -> Multiport Switch2/8, Multiport Switch2/7, Multiport Switch2/4, Multiport Switch2/3, Multiport Switch2/2
  [ON] -> Multiport Switch2/6, Multiport Switch2/5
  [SCCmmState] -> Multiport Switch2/1
  [SCCmmState] -> Multiport Switch1/1
  OFF/1 -> Multiport Switch1/2, [OFF]
  Multiport Switch1/1 -> MainModeACC_CAN/1  "MainModeACC_CAN"
  ON/1 -> Multiport Switch1/8, Multiport Switch1/7, Multiport Switch1/6, Multiport Switch1/5, Multiport Switch1/4, Multiport Switch1/3, [ON]
  Constant1/1 -> ACCFailInfo_CAN/1  "ACCFailInfo_CAN"
  Compare To Constant2/1 -> Switch9/2
  Constant8/1 -> Switch9/1
  Switch9/1 -> AliveCounterACC_CAN/1, Memory/1  "AliveCounterACC_CAN"
  Memory/1 -> Compare To Constant2/1, Add2/1  "AliveCounterACC_CAN_Old"
  Add2/1 -> Switch9/3
  Constant9/1 -> Add2/2
  aReq/1 -> aReqMax_CAN/1, aReqMin_CAN/1
  uiHeadwayState/1 -> Switch1/3, Relational Operator8/2
  HEADWAY_STATE_4/1 -> Relational Operator8/1
  [OFF] -> PreFill_CAN/1
  Multiport Switch4/1 -> ObjValid_CAN/1  "ObjValid_CAN"
  Constant3/1 -> DriverAlertDisplay_CAN/1
  Constant2/1 -> TakeOverReq_CAN/1
  NODISPLAY_CANSPEC/1 -> Multiport Switch3/8, Multiport Switch3/5, Multiport Switch3/3, Multiport Switch3/2, Multiport Switch3/4, Multiport Switch3/7
  Multiport Switch/1 -> ACCMode_CAN/1  "ACCMode_CAN"
  SHUTOFF_CANSPEC/1 -> Multiport Switch/8
  OVERRIDE_CANSPEC/1 -> Multiport Switch/7
  ENGAGED_CANSPEC/1 -> Multiport Switch/6, Multiport Switch/5, Multiport Switch/4
  [OFF] -> Multiport Switch/3, Multiport Switch/2
  SCCmmState/1 -> [SCCmmState], Multiport Switch/1  "SCCmmState"

== system Control_test/OutputProcessing/ACC_Interface/SCC2 Processing ==
  spObjValid : Inport
  spClearance : Inport  Port=2
  spRelSpdCalMps : Inport  Port=3
  OFF : Constant  Value=0  SampleTime=0.02
  Rate Transition{,1..3} (4 alike) : RateTransition  OutPortSampleTime=0.02
  Rate Transition{4..7} (4 alike) : RateTransition  OutPortSampleTime=0.01
  ACC_ObjLatPos_CAN : Outport
  ACC_ObjDist_CAN : Outport  Port=2
  ACC_ObjRelSpd_CAN : Outport  Port=3
  ACC_ObjStatus_CAN : Outport  Port=4
  wires:
  spObjValid/1 -> Rate Transition4/1
  OFF/1 -> Rate Transition5/1
  spClearance/1 -> Rate Transition6/1
  spRelSpdCalMps/1 -> Rate Transition7/1
  Rate Transition/1 -> ACC_ObjStatus_CAN/1
  Rate Transition1/1 -> ACC_ObjLatPos_CAN/1
  Rate Transition2/1 -> ACC_ObjDist_CAN/1
  Rate Transition3/1 -> ACC_ObjRelSpd_CAN/1
  Rate Transition4/1 -> Rate Transition/1
  Rate Transition5/1 -> Rate Transition1/1
  Rate Transition6/1 -> Rate Transition2/1
  Rate Transition7/1 -> Rate Transition3/1

== system Control_test/OutputProcessing/RadarCanProcessing/Transmit Radar Msg 0x4F0 ==
  ipVehSpdWhl[m/s] : Inport
  ipSftLvrDFlag : Inport  Port=2
  ipYawRate[deg/s] : Inport  Port=3
  Constant2 : Constant  SampleTime=Inf
  Constant3 : Constant  Value=0  SampleTime=Inf
  Constant4 : Constant  SampleTime=Inf
  Gain : Gain  Gain=-1
  If : If  NumInputs=2  IfExpression=u1>=0 & u2==1
  If Action Subsystem : Subsystem  TreatAsAtomicUnit=on
  If Action Subsystem1 : Subsystem  TreatAsAtomicUnit=on
  Merge : Merge
  flag_direct : Gain
  CAN_RX_VEHICLE_SPEED : Outport
  CAN_RX_VEHICLE_SPEED_DIRECTION : Outport  Port=2
  CAN_RX_YAW_RATE : Outport  Port=3
  CAN_RX_YAW_RATE_VALIDITY : Outport  Port=4
  wires:
  Gain/1 -> CAN_RX_YAW_RATE/1  "CAN_RX_YAW_RATE"
  ipYawRate[deg/s]/1 -> Gain/1
  ipSftLvrDFlag/1 -> If/2
  Merge/1 -> flag_direct/1
  Constant4/1 -> If Action Subsystem1/1(In1)
  Constant3/1 -> If Action Subsystem/1(In1)
  If/2 -> If Action Subsystem1/Action
  If Action Subsystem1/1(Out1) -> Merge/2
  If Action Subsystem/1(Out1) -> Merge/1
  If/1 -> If Action Subsystem/Action
  ipVehSpdWhl[m/s]/1 -> If/1, CAN_RX_VEHICLE_SPEED/1  "CAN_RX_VEHICLE_SPEED"
  Constant2/1 -> CAN_RX_YAW_RATE_VALIDITY/1  "CAN_RX_YAW_RATE_VALIDITY"
  flag_direct/1 -> CAN_RX_VEHICLE_SPEED_DIRECTION/1

== system Control_test/OutputProcessing/RadarCanProcessing/Transmit Radar Msg 0x4F1 ==
  Constant1 : Constant  Value=64  SampleTime=Inf
  Constant2 : Constant  Value=0  SampleTime=Inf
  Constant3 : Constant  Value=0.33  SampleTime=Inf
  Constant4 : Constant  SampleTime=Inf
  Constant5 : Constant  SampleTime=Inf
  CAN_RX_LATERAL_MOUNTING_OFFSET : Outport
  CAN_RX_MAXIMUM_TRACKS : Outport  Port=2
  CAN_RX_RADAR_CMD_RADIATE : Outport  Port=3
  CAN_RX_MMR_UPSIDE_DOWN : Outport  Port=4
  CAN_RX_VEHICLE_SPEED_VALIDITY : Outport  Port=5
  wires:
  Constant5/1 -> CAN_RX_VEHICLE_SPEED_VALIDITY/1  "CAN_RX_VEHICLE_SPEED_VALIDITY"
  Constant1/1 -> CAN_RX_MAXIMUM_TRACKS/1  "CAN_RX_MAXIMUM_TRACKS"
  Constant2/1 -> CAN_RX_MMR_UPSIDE_DOWN/1  "CAN_RX_MMR_UPSIDE_DOWN"
  Constant3/1 -> CAN_RX_LATERAL_MOUNTING_OFFSET/1  "CAN_RX_LATERAL_MOUNTING_OFFSET"
  Constant4/1 -> CAN_RX_RADAR_CMD_RADIATE/1  "CAN_RX_RADAR_CMD_RADIATE"

== system Control_test/OutputProcessing/RadarCanProcessing/Transmit Radar Msg 0x5F2 ==
  Constant1 : Constant  Value=90  SampleTime=Inf
  Constant2 : Constant  SampleTime=Inf
  Constant3 : Constant  Value=20  SampleTime=Inf
  Constant4 : Constant  Value=0  SampleTime=Inf
  Constant5 : Constant  Value=2000  SampleTime=Inf
  Constant6 : Constant  Value=0  SampleTime=Inf
  Constant7 : Constant  Value=0  SampleTime=Inf
  Constant8 : Constant  Value=250  SampleTime=Inf
  CAN_RX_RADAR_FOV_LR : Outport
  CAN_RX_RADAR_FOV_MR : Outport  Port=2
  CAN_RX_AUTO_ALIGN_DISABLE : Outport  Port=3
  CAN_RX_AUTO_ALIGN_CONVERGED : Outport  Port=4
  CAN_RX_AALIGN_AVG_CTR_TOTAL : Outport  Port=5
  CAN_RX_SERV_ALIGN_ENABLE : Outport  Port=6
  CAN_RX_SERV_ALIGN_TYPE : Outport  Port=7
  CAN_RX_SERV_ALIGN_UPDATES_NEED : Outport  Port=8
  wires:
  Constant8/1 -> CAN_RX_SERV_ALIGN_UPDATES_NEED/1  "CAN_RX_SERV_ALIGN_UPDATES_NEED"
  Constant7/1 -> CAN_RX_SERV_ALIGN_TYPE/1  "CAN_RX_SERV_ALIGN_TYPE"
  Constant6/1 -> CAN_RX_SERV_ALIGN_ENABLE/1  "CAN_RX_SERV_ALIGN_ENABLE"
  Constant4/1 -> CAN_RX_AUTO_ALIGN_DISABLE/1  "CAN_RX_AUTO_ALIGN_DISABLE"
  Constant3/1 -> CAN_RX_RADAR_FOV_LR/1  "CAN_RX_RADAR_FOV_LR"
  Constant2/1 -> CAN_RX_AUTO_ALIGN_CONVERGED/1  "CAN_RX_AUTO_ALIGN_CONVERGED"
  Constant1/1 -> CAN_RX_RADAR_FOV_MR/1  "CAN_RX_RADAR_FOV_MR"
  Constant5/1 -> CAN_RX_AALIGN_AVG_CTR_TOTAL/1  "CAN_RX_AALIGN_AVG_CTR_TOTAL"

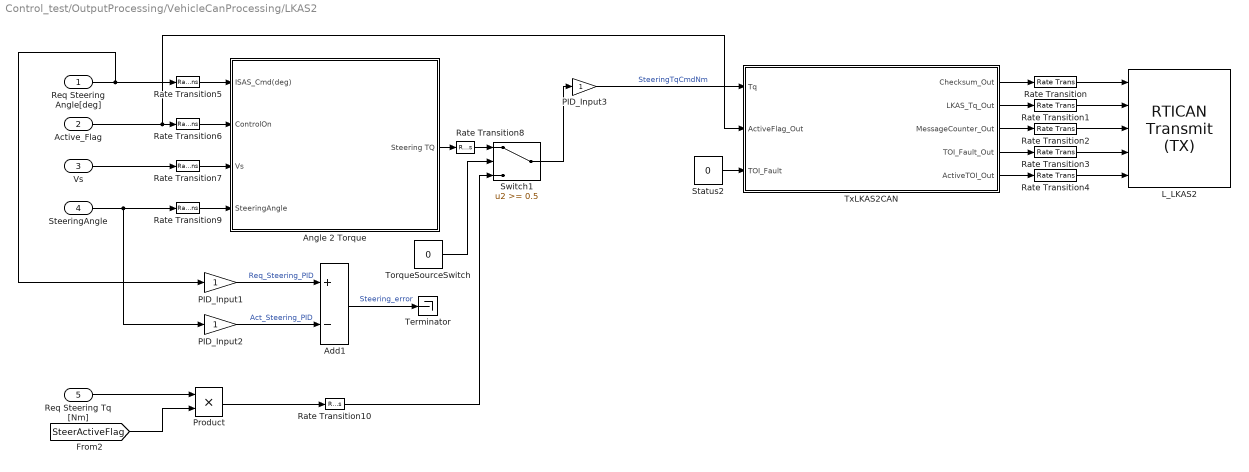
== system Control_test/OutputProcessing/VehicleCanProcessing/LKAS2 ==
  Req Steering Angle[deg] : Inport
  Active_Flag : Inport  Port=2
  Vs : Inport  Port=3
  SteeringAngle : Inport  Port=4
  Req Steering Tq [Nm] : Inport  Port=5
  Add1 : Sum  Inputs=+-
  Angle 2 Torque : Subsystem  TreatAsAtomicUnit=on  SystemSampleTime=0.01
  L_LKAS2 : rtican/RTICAN Transmit (TX)   Reserved1=[]  Reserved2=[]  Reserved3=[]  Reserved4=[]  SfcnMessage=[]  Msg_Struct=[]  BoardTypeNo=[]  BoardNo=[]  ChannelNo=[]  Parameters=[]  DialogFcn=[]  UnitName=[]  Revision=[]  UnitValues=[]  DSProperties=struct('RTI',struct('Version',uint32(5),'BlockType',struct('isSLSource',uint8(1),'isSLSink',uint8(1),'isHWSource',uint8(0),'isHWSink',uint8(0),'isSetup',uint8(0),'isInline',uint8(1),'isNonInline',uint8(0),'isInterrupt',uint8(0),'isChannelwise',uint8(0)),'IOBoardType','RTICAN','UnitType','MESSAGE','Identifier','TX','DialogType','MSVC','BlockSet','RTICAN','SlaveProcessor','CAN'))  RTIBlockInterface=struct('InputPortsWidth',int32([1 1 1 1 1]),'InputPortsActive',[1 1 1 1 1],'InputPortsName',{{'CF_Lkas_Chksum2','CR_Lkas_StrToqReq','CF_Lkas_MsgCount2','CF_Lkas_ToiFlt','CF_Lkas_ActToi'}},'InputPortsDataType',{{'SS_DOUBLE','SS_DOUBLE','SS_DOUBLE','SS_DOUBLE','SS_DOUBLE'}},'OutputPortsWidth',int32(0),'OutputPortsActive',0,'OutputPortsName',{{''}},'DialogFcn','rtican_message_interface_gui','BlockDisplay',{{'','center'}},'IconTransparency','on','InitLevel',3,'BlockName',struct('Token',{{'L_LKAS2'}}),'SampleTime',{{0.01}},'TriggerPort',{{'none'}},'EnablePort',{{'none'}})  RTIBlockParameters=struct('BoardTypeNo',{{1,'OFF',[]}},'BoardNo',{{1,'ON',[1 16]}},'ChannelNo',{{1,'ON',[1 2]}},'Parameters',{{struct('DataFileSupport',struct('DataFileSelectedMaster',1,'DataFileSelectedLocal',1,'DataFileName',['c:\users\mpc\dropbox\hyundai car setup\hmc_can_for_ucb_v1.dbc|c:\users\mpc\dropbox\hyundai car setup\mobileye spec new\mobileye_mando_camera_ucb_v2.dbc|'],'DataFileDate',['26-Nov-2014 10:54:28'],'SelectedFile','c:\users\mpc_car\documents\github\mpc-car\dbcfiles\hmc_can_for_ucb_v2.dbc','InterfaceFcn','rtican_dbc_file_parser'),'Options',struct('StatusSelected',0,'TimeSelected',0,'DeltaTimeSelected',0,'DelayTimeSelected',0,'DelayTimeTXCommandSelected',0,'EncodeSetUnusedBitsToOne',0,'EnableMsgLoopback',0,'TriggerPort',struct('Selected',0,'TriggerType',0),'EnablePortSelected',0,'SignalOnPortnameSelected',1,'UserCoding',struct('Selected',0,'InterfaceFile','UserEncodingFile','FcnName','UserEncodeFcn','InportSelected',0,'InportWidth',1,'OutportSelected',0,'OutportWidth',1),'TerminationMsg',struct('Selected',0,'Byte0_7','0'),'InitialMsg',struct('Selected',0,'Byte0_7','0')),'Message',struct('MsgOnBlocknameSelected',1,'MsgName','L_LKAS2','MsgIdFormat',0,'MsgId',258,'MsgLength',4,'NumSignals',5,'SampleTime',0.01,'StartTime',struct('Selected',0,'Value',0),'AutoRepeatTime',struct('Selected',0,'Value',0.1),'Timeout',struct('Selected',0,'Value',0.1),'DelayTime',struct('Selected',0,'Value',0.1),'Signal',struct('SgnName',{'CF_Lkas_Chksum2','CR_Lkas_StrToqReq','CF_Lkas_MsgCount2','CF_Lkas_ToiFlt','CF_Lkas_ActToi'},'SgnStartBit',{0,8,19,23,31},'SgnLength',{8,11,4,1,1},'ByteLayout',{0,0,0,0,0},'Factor',{1,0.0078125,1,1,1},'Offset',{0,-8,0,0,0},'SgnComment',{'','','','',''},'SgnUnit',{'','Nm','','',''},'Min',{0,-8,0,0,0},'Max',{255,8,15,1,1},'SgnType',{0,0,0,0,0},'SLDataType',{'SS_DOUBLE','SS_DOUBLE','SS_DOUBLE','SS_DOUBLE','SS_DOUBLE'},'DataType',{0,0,0,0,0},'ModeValue',{-1,-1,-1,-1,-1}),'MsgIdNumFormat',0,'MsgComment',{{''}}),'Version',1.2,'general',struct('isFromLib',0)),'OFF',[]}},'GroupId',{{struct('Group',{{'RTICAN'}},'No',1,'Behavior',{{'NAMECHANGE'}},'BlockType',{{'SINK'}},'NameChangeFlag',0),'OFF',[]}},'SFcnRTICANMessage',{{struct('MsgType','TX','SFcnPortType','Scalar','MsgName','L_LKAS2','MsgIdFormat','STD','MsgId',258,'MsgLength',4,'NumSignals',5,'SampleTime',0.01,'StartTime',struct('Selected','no','Value',0),'AutoRepeatTime',struct('Selected','no','Value',0.1),'Timeout',struct('Selected','no','Value',0.1),'Signal',struct('SgnName',{'CF_Lkas_Chksum2','CR_Lkas_StrToqReq','CF_Lkas_MsgCount2','CF_Lkas_ToiFlt','CF_Lkas_ActToi'},'SgnStartBit',{0,8,19,23,31},'SgnLength',{8,11,4,1,1},'ByteLayout',{['little endian'],['little endian'],['little endian'],['little endian'],['little endian']},'Factor',{1,0.0078125,1,1,1},'Offset',{0,-8,0,0,0},'SgnType',{'standard','standard','standard','standard','standard'},'SLDataType',{'SS_DOUBLE','SS_DOUBLE','SS_DOUBLE','SS_DOUBLE','SS_DOUBLE'},'DataType',{['unsigned int'],['unsigned int'],['unsigned int'],['unsigned int'],['unsigned int']},'ModeValue',{-1,-1,-1,-1,-1}),'StatusSelected','no','TimeSelected','no','DeltaTimeSelected','no','DelayTimeSelected','no','DelayTimeTXCommandSelected','no','EncodeSetUnusedBitsToOne','no','EnableMsgLoopback','no','TriggerPort',struct('Selected','no','TriggerType',0),'EnablePortSelected','no','UserCoding',struct('Selected','no','InterfaceFile','UserEncodingFile','FcnName','UserEncodeFcn','InportSelected','no','InportWidth',1,'OutportSelected','no','OutportWidth',1),'TerminationMsg',struct('Selected','no','Byte0','0x00','Byte1','0x00','Byte2','0x00','Byte3','0x00','Byte4','0x00','Byte5','0x00','Byte6','0x00','Byte7','0x00'),'InitialMsg',struct('Selected','no','Byte0','0x00','Byte1','0x00','Byte2','0x00','Byte3','0x00','Byte4','0x00','Byte5','0x00','Byte6','0x00','Byte7','0x00'),'BoardType','DS1','BoardNo',1,'ControllerNo',1),'OFF',[]}},'TLCFileName',{{'rtican_tx_message','OFF',[]}})  RTISFcnParameters=struct('SFcnRTICANMessage','struct','TLCFileName','char')  RTIBlockParaDefault=struct('BoardTypeNo',4302,'BoardNo',1,'ChannelNo',1,'Parameters',struct('DataFileSupport',struct('DataFileSelectedMaster',0,'DataFileSelectedLocal',0,'DataFileName','','DataFileDate','','SelectedFile',['<no file selected>']),'Options',struct('StatusSelected',1,'TimeSelected',1,'DeltaTimeSelected',1,'DelayTimeSelected',1,'DelayTimeTXCommandSelected',0,'EncodeSetUnusedBitsToOne',0,'EnableMsgLoopback',0,'TriggerPort',struct('Selected',0,'TriggerType','rising'),'EnablePortSelected',0,'SignalOnPortnameSelected',1,'UserCoding',struct('Selected',0,'InterfaceFile','UserEncodingFile','FcnName','UserEncodeFcn','InportSelected',0,'InportWidth',1,'OutportSelected',0,'OutportWidth',1),'TerminationMsg',struct('Selected',0,'Byte0_7','0'),'InitialMsg',struct('Selected',0,'Byte0_7','0')),'Message',struct('MsgOnBlocknameSelected',0,'MsgName',['TX Message'],'MsgIdFormat',0,'MsgId',100,'MsgLength',8,'NumSignals',1,'SampleTime',-1,'StartTime',struct('Selected',0,'Value',0),'AutoRepeatTime',struct('Selected',0,'Value',0.1),'Timeout',struct('Selected',0,'Value',0.1),'DelayTime',struct('Selected',0,'Value',0.1),'Signal',struct('SgnName',['TX signal'],'SgnStartBit',0,'SgnLength',8,'SgnType',0,'ModeValue',-1,'DataType',0,'SLDataType','SS_DOUBLE','ByteLayout',0,'Factor',1,'Offset',0,'Min',0,'Max',255,'SgnComment',{{}},'SgnUnit',''),'MsgIdNumFormat',0,'MsgComment',{{''}}),'Version',1.2,'general',struct('isFromLib',1)),'GroupId',struct('Group',{{'RTICAN'}},'No',1,'Behavior',{{'NAMECHANGE'}},'BlockType',{{'SINK'}},'NameChangeFlag',0),'SFcnRTICANMessage',struct('MsgType','TX','MsgName',['TX Message'],'MsgIdFormat','STD','MsgId',100,'MsgLength',2,'NumSignals',1,'SampleTime',-1,'StartTime',struct('Selected','no','Value',0),'AutoRepeatTime',struct('Selected','no','Value',0.1),'Timeout',struct('Selected','no','Value',0.1),'DelayTime',struct('Selected','no','Value',0.1),'Signal',struct('SgnName',['TX signal'],'SgnStartBit',0,'SgnLength',8,'SgnType','standard','ModeValue',-1,'DataType',['unsigned int'],'ByteLayout',['little endian'],'SLDataType','SS_DOUBLE','Factor',1,'Offset',0),'StatusSelected','yes','TimeSelected','yes','DeltaTimeSelected','yes','DelayTimeSelected','yes','EnablePortSelected','no','EnableMsgLoopback','no','DelayTimeTXCommandSelected','no','EncodeSetUnusedBitsToOne','no','UserCoding',struct('Selected','no','InterfaceFile','UserDecodingFile','FcnName','UserDecodeFcn','InportSelected','no','InportWidth',1,'OutportSelected','no','OutportWidth',1),'TerminationMsg',struct('Selected','no','Byte0','0x00','Byte1','0x00','Byte2','0x00','Byte3','0x00','Byte4','0x00','Byte5','0x00','Byte6','0x00','Byte7','0x00'),'InitialMsg',struct('Selected','no','Byte0','0x00','Byte1','0x00','Byte2','0x00','Byte3','0x00','Byte4','0x00','Byte5','0x00','Byte6','0x00','Byte7','0x00'),'TriggerPort',struct('Selected','no','TriggerType','rising'),'BoardType','DS4302','BoardNo',1,'ControllerNo',1,'SFcnPortType','Scalar'),'TLCFileName','rtican_tx_message')
      settings: AttributesFormatString=Group Id: RTICAN1\n
  PID_Input1 : Gain
  PID_Input2 : Gain
  PID_Input3 : Gain
  Product : Product
  Rate Transition{,1..4,6} (6 alike) : RateTransition  OutPortSampleTime=0.01
  Rate Transition10 : RateTransition  Deterministic=off  OutPortSampleTime=0.001
  Rate Transition5 : RateTransition  Integrity=off  OutPortSampleTime=0.01
  Rate Transition7 : RateTransition  Integrity=off  OutPortSampleTime=0.01
  Rate Transition8 : RateTransition  Deterministic=off  OutPortSampleTime=0.001
  Rate Transition9 : RateTransition  Integrity=off  OutPortSampleTime=0.01
  Status2 : Constant  Value=0
  Switch1 : Switch  Threshold=0.5
  Terminator : Terminator
  TorqueSourceSwitch : Constant  Value=0
  TxLKAS2CAN : Subsystem  TreatAsAtomicUnit=on
  wires:
  Status2/1 -> TxLKAS2CAN/3(TOI_Fault)
  Req Steering Angle[deg]/1 -> PID_Input1/1, Rate Transition5/1
  Active_Flag/1 -> TxLKAS2CAN/2(ActiveFlag_Out), Rate Transition6/1
  Vs/1 -> Rate Transition7/1
  SteeringAngle/1 -> Rate Transition9/1, PID_Input2/1
  Add1/1 -> Terminator/1  "Steering_error"
  PID_Input1/1 -> Add1/1  "Req_Steering_PID"
  PID_Input2/1 -> Add1/2  "Act_Steering_PID"
  Angle 2 Torque/1(Steering TQ) -> Rate Transition8/1
  Switch1/1 -> PID_Input3/1
  Rate Transition7/1 -> Angle 2 Torque/3(Vs)
  Rate Transition9/1 -> Angle 2 Torque/4(SteeringAngle)
  Rate Transition8/1 -> Switch1/1
  Rate Transition6/1 -> Angle 2 Torque/2(ControlOn)
  TxLKAS2CAN/1(Checksum_Out) -> Rate Transition/1
  TxLKAS2CAN/2(LKAS_Tq_Out) -> Rate Transition1/1
  TxLKAS2CAN/3(MessageCounter_Out) -> Rate Transition2/1
  TxLKAS2CAN/4(TOI_Fault_Out) -> Rate Transition3/1
  TxLKAS2CAN/5(ActiveTOI_Out) -> Rate Transition4/1
  Rate Transition/1 -> L_LKAS2/1
  Rate Transition1/1 -> L_LKAS2/2
  Rate Transition2/1 -> L_LKAS2/3
  Rate Transition3/1 -> L_LKAS2/4
  Rate Transition4/1 -> L_LKAS2/5
  Rate Transition5/1 -> Angle 2 Torque/1(ISAS_Cmd(deg))
  [SteerActiveFlag] -> Product/2
  Req Steering Tq [Nm]/1 -> Product/1
  TorqueSourceSwitch/1 -> Switch1/2
  Product/1 -> Rate Transition10/1
  Rate Transition10/1 -> Switch1/3
  PID_Input3/1 -> TxLKAS2CAN/1(Tq)  "SteeringTqCmdNm"

== system Control_test/RTI Data/RTI Data Store/RTI Data Store ==
  RTI Data Store : Subsystem  mask(RTI_DATA_STORE){}
      mask help:
      | RTI Data Store Block. This block is used by RTI to store internal model dependent data. Deleting this block will result in data loss.
      |
      | NEVER DELETE, COPY, OR MODIFY THIS BLOCK!
      mask Help:
      | RTI Data Store Block. This block is used by RTI to store internal model dependent data. Deleting this block will result in data loss.
      | 
      | NEVER DELETE, COPY, OR MODIFY THIS BLOCK!
      mask Display: text(0.5, 0.5, ' ', 'HorizontalAlignment', 'center');
